simulink model "closed"  (R2024a)
settings: Solver=VariableStepAuto  StartTime=0.0  StopTime=2  MaxStep=1e-4  RelTol=1e-4
values from neighbouring files (symbols this model uses):
  A = [8  1  11, ... (first row only)    [main1.m]
  B = [-1 -3 3]'    [main1.m]
  K = K_cell{i}    [graphics.m]    (also in main1.m)
  x0 = [1 1 1]'    [main1.m]
settings Model: Creator=eva  LastModifiedBy=eva

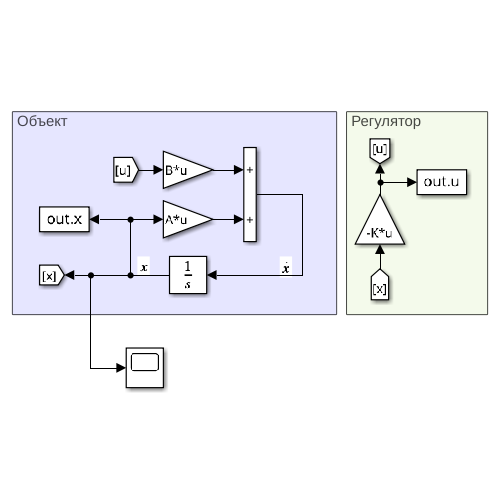
[thumbnail: Simulink's stored preview of the top-level diagram]
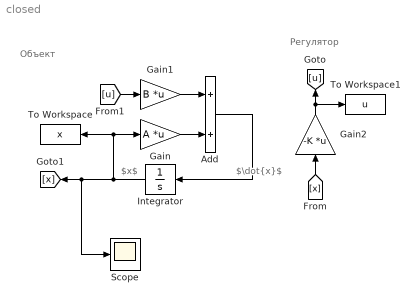
== system closed ==
  note: Регулятор
  note: Объект
  note: $\dot{x}$
  note: $x$
  Add : Sum
  Gain : Gain  Gain=A  Multiplication=Matrix(K*u)
  Gain1 : Gain  Gain=B  Multiplication=Matrix(K*u)
  Gain2 : Gain  Gain=-K  Multiplication=Matrix(K*u)
  Integrator : Integrator  InitialCondition=x0
  Scope : Scope
  To Workspace : ToWorkspace  VariableName=x  SaveFormat=Structure With Time  SampleTime=-1
  To Workspace1 : ToWorkspace  VariableName=u  SaveFormat=Structure With Time  SampleTime=-1
  wires:
  Gain1/1 -> Add/1
  Gain/1 -> Add/2
  Add/1 -> Integrator/1
  Integrator/1 -> Scope/1, [x], To Workspace/1, Gain/1
  Gain2/1 -> To Workspace1/1, [u]
  [x] -> Gain2/1
  [u] -> Gain1/1
